simulink library "lib_clarke_transform"  (R2023a)
settings: Solver=VariableStepAuto  StartTime=0.0  StopTime=10.0  RelTol=1e-3
libraries: lib_conversion x3
settings Model: Creator=cav2ofo  LastModifiedBy=xiaoqiang.yuan
settings OptimizationCC: ReuseModelBlockBuffer=off

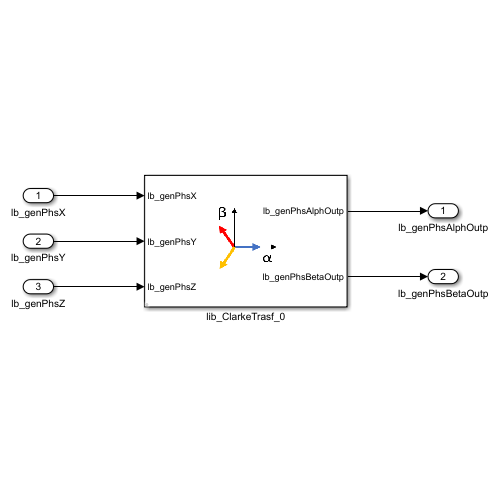
[thumbnail: Simulink's stored preview of the top-level diagram]
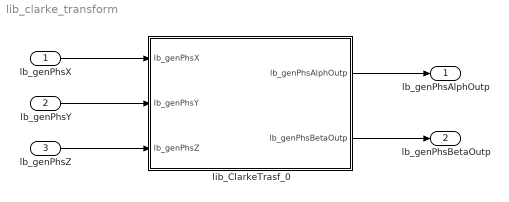
== system lib_clarke_transform ==
  lb_genPhsX : Inport
  lb_genPhsY : Inport  Port=2
  lb_genPhsZ : Inport  Port=3
  lib_ClarkeTrasf_0 : Subsystem  VariantControl=ClarkTransf_MIL_flo  mask{lb_parAccmDataType=fixdt(1,16,2^-6,0), lb_parUnBalcSys=off}
      mask prompts: lb_parAccmDataType "Accumulator data type:"; lb_parUnBalcSys "Unbalanced system"
      mask init:
      | if lb_parUnBalcSys
      |     set_param([gcb,'/vss_ClarkeTransform'],'LabelModeActiveChoice','lb_parUnBalcSysModeLbl');
      | else
      |     set_param([gcb,'/vss_ClarkeTransform'],'LabelModeActiveChoice','lb_parBalcSysModeLbl');
      | end
      mask DialogControl DescGroupVar Prompt: Clarke Transform
      mask DialogControl DescTextVar Prompt: VHIT Control Library
      mask DialogControl clarkeDesc Prompt: This block performs Clarke transform on the input signals. You can choose the computation logic either for symmetric or asymmetric motor type.
      mask DialogControl dataTypDesc Prompt: Data type
      mask DialogControl Control4 Prompt: The accumulator data type shall be defined considering the value that is two times the value of input signal.
      mask DialogControl operMod Prompt: Operating modes
      mask DialogControl Control2 Prompt: By default the computation for symmetric motor is performed. Tick the following check box for asymmetric motor type.
      mask Display: image('ClarkTransf.png'); % Use "Edit Image" on toolstrip to change.
  lb_genPhsAlphOutp : Outport
  lb_genPhsBetaOutp : Outport  Port=2
  wires:
  lb_genPhsX/1 -> lib_ClarkeTrasf_0/1(lb_genPhsX)
  lb_genPhsY/1 -> lib_ClarkeTrasf_0/2(lb_genPhsY)
  lb_genPhsZ/1 -> lib_ClarkeTrasf_0/3(lb_genPhsZ)
  lib_ClarkeTrasf_0/1(lb_genPhsAlphOutp) -> lb_genPhsAlphOutp/1
  lib_ClarkeTrasf_0/2(lb_genPhsBetaOutp) -> lb_genPhsBetaOutp/1

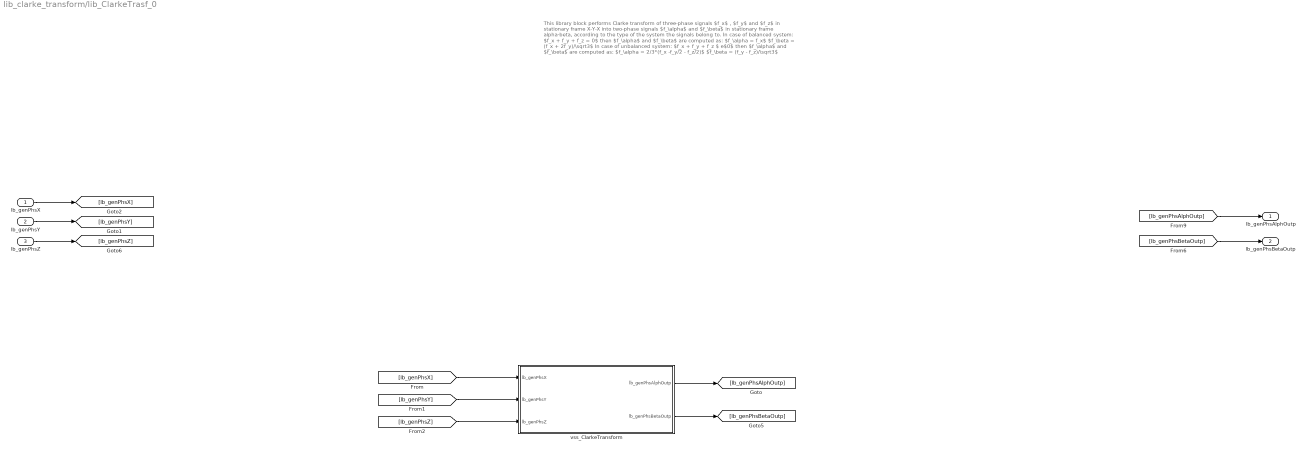
== system lib_clarke_transform/lib_ClarkeTrasf_0 ==
  note: This library block performs Clarke transform of three-phase signals $f_x$ , $f_y$ and $f_z$
      | in stationary frame X-Y-X into two-phase signals $f_\alpha$ and $f_\beta$ in stationary frame alpha-beta,
      | according to the type of the system the signals belong to.
      | In case of balanced system:
      | $f_x + f_y + f_z = 0$
      | then $f_\alpha$ and $f_\beta$ are computed as:
      | $f_\alpha = f_x$
      | $f_\beta = (f_x + 2f_y)/\sqrt3$
      | In case of unbalanced system:
      | $f_x + f_y + f_z $\ne$0$
      | then $f_\alpha$ and $f_\beta$ are computed as:
      | $f_\alpha = 2/3*(f_x -f_y/2 - f_z/2)$
      | $f_\beta = (f_y - f_z)/\sqrt3$
  lb_genPhsX : Inport
  lb_genPhsY : Inport  Port=2
  lb_genPhsZ : Inport  Port=3
  vss_ClarkeTransform : Subsystem  Variant=on  VariantControlMode=label  LabelModeActiveChoice=lb_parBalcSysModeLbl
  lb_genPhsAlphOutp : Outport  VectorParamsAs1DForOutWhenUnconnected=off
  lb_genPhsBetaOutp : Outport  Port=2  VectorParamsAs1DForOutWhenUnconnected=off
  wires:
  [lb_genPhsBetaOutp] -> lb_genPhsBetaOutp/1
  [lb_genPhsAlphOutp] -> lb_genPhsAlphOutp/1
  lb_genPhsX/1 -> [lb_genPhsX]
  lb_genPhsY/1 -> [lb_genPhsY]
  lb_genPhsZ/1 -> [lb_genPhsZ]
  [lb_genPhsX] -> vss_ClarkeTransform/1(lb_genPhsX)
  [lb_genPhsY] -> vss_ClarkeTransform/2(lb_genPhsY)
  [lb_genPhsZ] -> vss_ClarkeTransform/3(lb_genPhsZ)
  vss_ClarkeTransform/1(lb_genPhsAlphOutp) -> [lb_genPhsAlphOutp]
  vss_ClarkeTransform/2(lb_genPhsBetaOutp) -> [lb_genPhsBetaOutp]

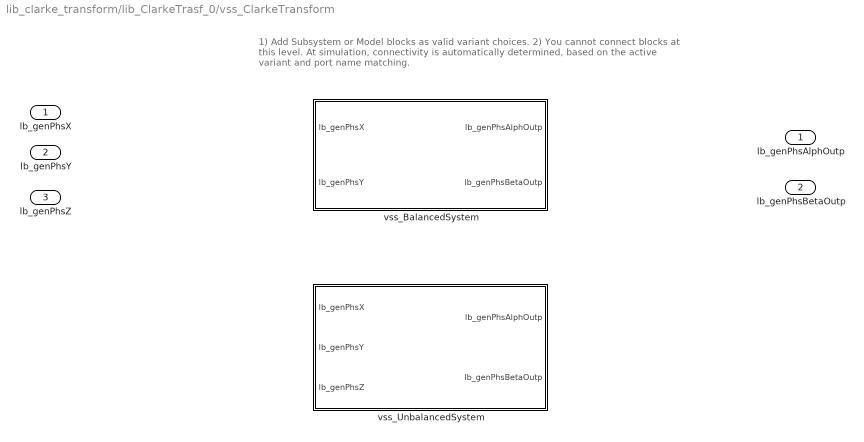
== system lib_clarke_transform/lib_ClarkeTrasf_0/vss_ClarkeTransform ==
  note: 1) Add Subsystem or Model blocks as valid variant choices.
      | 2) You cannot connect blocks at this level. At simulation, connectivity is automatically
      | determined, based on the active variant and port name matching.
  lb_genPhsX : Inport
  lb_genPhsY : Inport  Port=2
  lb_genPhsZ : Inport  Port=3
  vss_BalancedSystem : Subsystem  VariantControl=lb_parBalcSysModeLbl
  vss_UnbalancedSystem : Subsystem  VariantControl=lb_parUnBalcSysModeLbl
  lb_genPhsAlphOutp : Outport
  lb_genPhsBetaOutp : Outport  Port=2

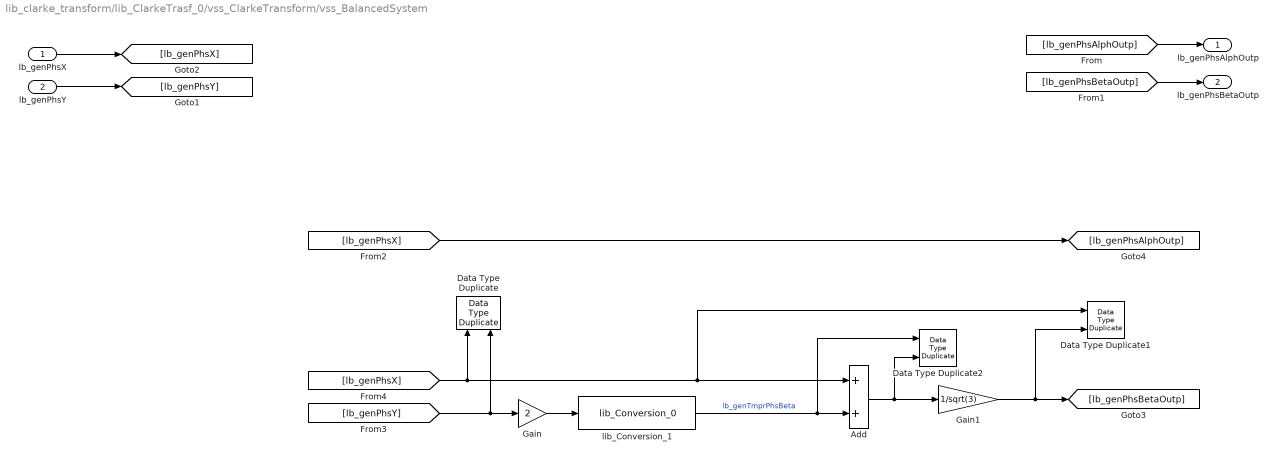
== system lib_clarke_transform/lib_ClarkeTrasf_0/vss_ClarkeTransform/vss_BalancedSystem ==
  lb_genPhsX : Inport
  lb_genPhsY : Inport  Port=2
  Add : Sum  OutDataTypeStr=Inherit: Inherit via back propagation  RndMeth=Simplest
  Data Type Duplicate : DataTypeDuplicate
  Data Type Duplicate1 : DataTypeDuplicate
  Data Type Duplicate2 : DataTypeDuplicate
  Gain : Gain  Gain=2  OutDataTypeStr=Inherit: Inherit via back propagation  RndMeth=Simplest
  Gain1 : Gain  Gain=1/sqrt(3)  OutDataTypeStr=Inherit: Inherit via back propagation  RndMeth=Simplest
  lib_Conversion_1 : lib_conversion/lib_Conversion_0  lb_parDataType=lb_parAccmDataType  lb_parOutpMaxVal=[]  lb_parOutpMinVal=[]  lb_parSatFlag=off
  lb_genPhsAlphOutp : Outport  VectorParamsAs1DForOutWhenUnconnected=off
  lb_genPhsBetaOutp : Outport  Port=2  VectorParamsAs1DForOutWhenUnconnected=off
  wires:
  [lb_genPhsBetaOutp] -> lb_genPhsBetaOutp/1
  Gain1/1 -> Data Type Duplicate1/2, [lb_genPhsBetaOutp]
  [lb_genPhsAlphOutp] -> lb_genPhsAlphOutp/1
  [lb_genPhsY] -> Data Type Duplicate/2, Gain/1
  lb_genPhsX/1 -> [lb_genPhsX]
  [lb_genPhsX] -> Data Type Duplicate/1, Add/1, Data Type Duplicate1/1
  lib_Conversion_1/1 -> Add/2, Data Type Duplicate2/1  "lb_genTmprPhsBeta"
  Gain/1 -> lib_Conversion_1/1
  [lb_genPhsX] -> [lb_genPhsAlphOutp]
  Add/1 -> Gain1/1, Data Type Duplicate2/2
  lb_genPhsY/1 -> [lb_genPhsY]

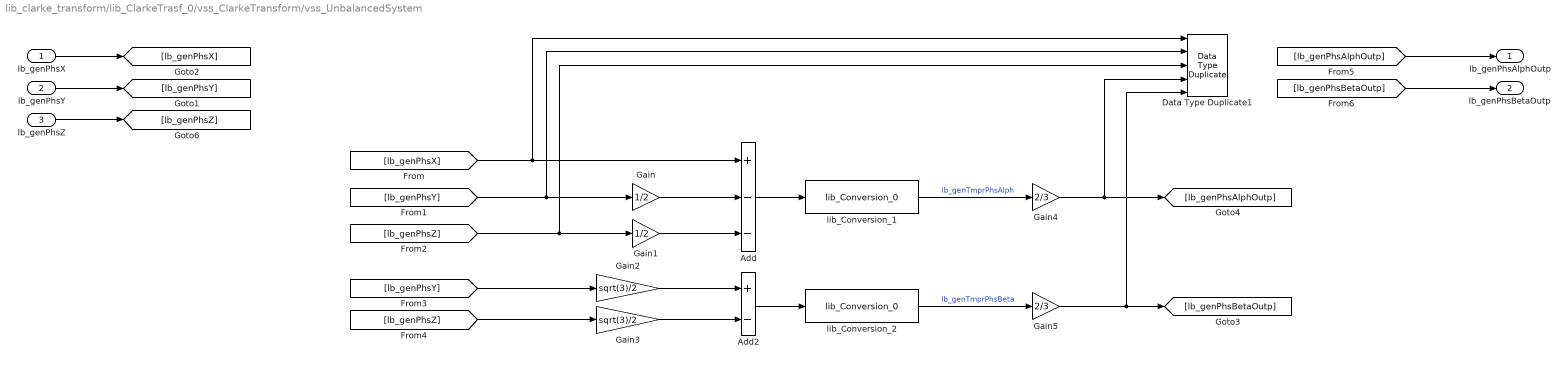
== system lib_clarke_transform/lib_ClarkeTrasf_0/vss_ClarkeTransform/vss_UnbalancedSystem ==
  lb_genPhsX : Inport
  lb_genPhsY : Inport  Port=2
  lb_genPhsZ : Inport  Port=3
  Add : Sum  Inputs=+--  InputSameDT=on  OutDataTypeStr=Inherit: Inherit via back propagation  RndMeth=Simplest  SaturateOnIntegerOverflow=on
  Add2 : Sum  Inputs=+-  InputSameDT=on  OutDataTypeStr=Inherit: Inherit via back propagation  RndMeth=Simplest  SaturateOnIntegerOverflow=on
  Data Type Duplicate1 : DataTypeDuplicate  NumInputPorts=5
  Gain : Gain  Gain=1/2  RndMeth=Simplest  OutDataTypeStr=Inherit: Same as input
  Gain1 : Gain  Gain=1/2  RndMeth=Simplest  OutDataTypeStr=Inherit: Same as input
  Gain2 : Gain  Gain=sqrt(3)/2  RndMeth=Simplest  OutDataTypeStr=Inherit: Same as input
  Gain3 : Gain  Gain=sqrt(3)/2  RndMeth=Simplest  OutDataTypeStr=Inherit: Same as input
  Gain4 : Gain  Gain=2/3  OutDataTypeStr=Inherit: Inherit via back propagation  RndMeth=Simplest
  Gain5 : Gain  Gain=2/3  OutDataTypeStr=Inherit: Inherit via back propagation  RndMeth=Simplest
  lib_Conversion_1 : lib_conversion/lib_Conversion_0  lb_parDataType=lb_parAccmDataType  lb_parOutpMaxVal=[]  lb_parOutpMinVal=[]  lb_parSatFlag=off
  lib_Conversion_2 : lib_conversion/lib_Conversion_0  lb_parDataType=lb_parAccmDataType  lb_parOutpMaxVal=[]  lb_parOutpMinVal=[]  lb_parSatFlag=off
  lb_genPhsAlphOutp : Outport  VectorParamsAs1DForOutWhenUnconnected=off
  lb_genPhsBetaOutp : Outport  Port=2  VectorParamsAs1DForOutWhenUnconnected=off
  wires:
  [lb_genPhsY] -> Gain2/1
  Add2/1 -> lib_Conversion_2/1
  [lb_genPhsX] -> Add/1, Data Type Duplicate1/1
  Gain/1 -> Add/2
  Add/1 -> lib_Conversion_1/1
  [lb_genPhsY] -> Gain/1, Data Type Duplicate1/2
  Gain3/1 -> Add2/2
  Gain4/1 -> Data Type Duplicate1/4, [lb_genPhsAlphOutp]
  Gain2/1 -> Add2/1
  [lb_genPhsZ] -> Gain3/1
  [lb_genPhsZ] -> Data Type Duplicate1/3, Gain1/1
  Gain5/1 -> Data Type Duplicate1/5, [lb_genPhsBetaOutp]
  Gain1/1 -> Add/3
  lb_genPhsY/1 -> [lb_genPhsY]
  lib_Conversion_2/1 -> Gain5/1  "lb_genTmprPhsBeta"
  lb_genPhsZ/1 -> [lb_genPhsZ]
  [lb_genPhsAlphOutp] -> lb_genPhsAlphOutp/1
  lib_Conversion_1/1 -> Gain4/1  "lb_genTmprPhsAlph"
  lb_genPhsX/1 -> [lb_genPhsX]
  [lb_genPhsBetaOutp] -> lb_genPhsBetaOutp/1
